simulink model "pneumatic_tank_models"  (R2018b)
settings: Solver=ode15s  StartTime=0.0  StopTime=60  FixedStep=1e-3  RelTol=1e-3
PreLoadFcn:
  | delta_p = 0.6; % MPa
  | p_init = 0.101325; % MPa
  | T_init = 293.15; % K
  | T_atm = 293.15; % K
  | 
  | A_valve_max = 4e-6; % m^2
  | A_valve_min = 1e-10; % m^2
  | 
  | A_pipe = 5e-6; % m^2
  | L_pipe = 1; % m
  | 
  | A_piston = 0.002; % m^2
  | L_piston = 0.2; % m
values from neighbouring files (symbols this model uses):
  a0 = a01    [sysid_tank.m]
  a1 = a11    [sysid_tank.m]
  a_lin = theta_lin_LS(1)    [sysid_tank.m]
  k_lin = theta_lin_LS(2)    [sysid_tank.m]
  p0 = 0.5*delta_p    (= 2.5)    [sysid_tank.m]
libraries: simulink x1
CloseFcn:
  | try,close(h1_ssc_pneumatic_actuator),end
  | clear h1_ssc_pneumatic_actuator
  | try,close(h2_ssc_pneumatic_actuator),end
  | clear h2_ssc_pneumatic_actuator
  | 
  | clear simlog_ssc_pneumatic_actuator tout
  | clear delta_p p_init T_init T_atm
  | clear A_valve_max A_valve_min
  | clear A_pipe L_pipe A_piston L_piston load
Description:
  | Pneumatic Actuation Circuit
  | 
  | Copyright 2016-2018 The MathWorks, Inc.
settings Model: Creator=MathWorks  LastModifiedBy=kjartan
settings DebuggingCC: LibraryContextMissingDiagnostic=none
settings SFSimCC: SimUseLocalCustomCode=off
settings RTWCC: RTWUseLocalCustomCode=off
settings CodeAppCC: StateflowObjectComments=on
settings GRTTargetCC: TargetLangStandard=C89/C90 (ANSI)
settings ConfigComp: CovMetricSettings=dsw  CovHtmlReporting=on  CovSaveCumulativeToWorkspaceVar=on  CovSaveSingleToWorkspaceVar=on  CovShowResultsExplorer=off  CovExternalEMLEnable=off
settings SimscapeCC: SimscapeNominalValues="[{\"value\":\"1\",\"unit\":\"A\"},{\"value\":\"1\",\"unit\":\"bar\"},{\"value\":\"1\",\"unit\":\"cm^2\"},{\"value\":\"1\",\"unit\":\"cm^3/s\"},{\"value\":\"500\",\"unit\":\"kJ/kg\"},{\"value\":\"1\",\"unit\":\"kW\"},{\"value\":\"1\",\"unit\":\"l\"},{\"value\":\"1\",\"unit\":\"N\"},{\"value\":\"1\",\"unit\":\"N*m\"},{\"value\":\"1\",\"unit\":\"V\"}]"  SimscapeLogType=all  SimscapeLogSimulationStatistics=on  SimscapeLogName=simlog_ssc_pneumatic_actuator  SimscapeLogDataHistory=10000

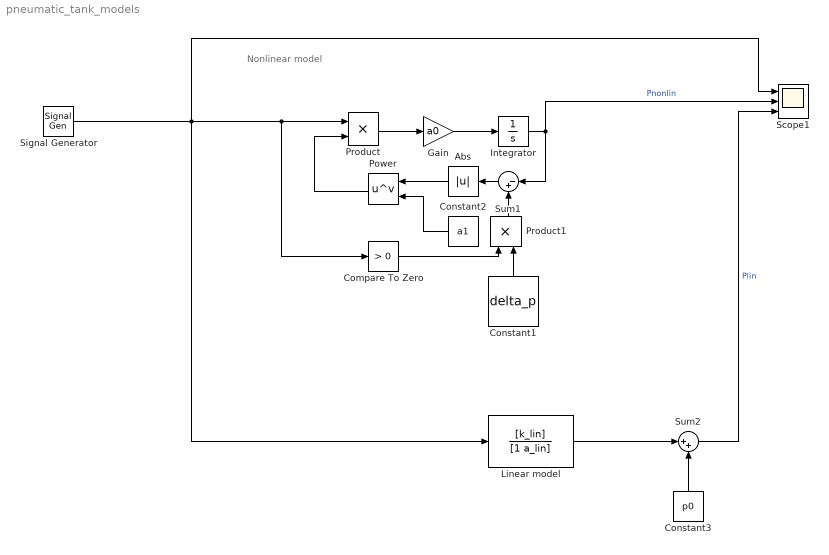
== system pneumatic_tank_models ==
  note: Nonlinear model
  Abs : Abs
  Compare To Zero : simulink/Logic and Bit Operations/Compare To Zero  relop=>  OutDataTypeStr=boolean
  Constant1 : Constant  Value=delta_p
  Constant2 : Constant  Value=a1
  Constant3 : Constant  Value=p0
  Gain : Gain  Gain=a0
  Integrator : Integrator  InitialCondition=p0
  Linear model : TransferFcn  Numerator=[k_lin]  Denominator=[1 a_lin]
  Power : Math  Operator=pow  SaturateOnIntegerOverflow=on
  Product : Product
  Product1 : Product
  Scope1 : Scope  NumInputPorts=3
  Signal Generator : SignalGenerator  WaveForm=square  Amplitude=2  Frequency=0.2  Units=rad/sec
  Sum1 : Sum  Inputs=|-+
  Sum2 : Sum  Inputs=|++
  wires:
  Signal Generator/1 -> Scope1/1, Linear model/1, Compare To Zero/1, Product/1
  Integrator/1 -> Sum1/1, Scope1/2  "Pnonlin"
  Compare To Zero/1 -> Product1/1
  Product1/1 -> Sum1/2
  Constant1/1 -> Product1/2
  Sum1/1 -> Abs/1
  Abs/1 -> Power/1
  Power/1 -> Product/2
  Constant2/1 -> Power/2
  Product/1 -> Gain/1
  Gain/1 -> Integrator/1
  Linear model/1 -> Sum2/1
  Constant3/1 -> Sum2/2
  Sum2/1 -> Scope1/3  "Plin"
